simulink model "motor1"  (R2022b)
settings: Solver=ode45  StartTime=0.0  StopTime=5  MaxStep=0.0001  RelTol=1e-3
values from neighbouring files (symbols this model uses):
  Beq = 1.26e-6    (= 1.26e-06)    [ex1.m]    (also in ex2.m)
  Jeq = mot.J + mld.J / gbox.N^2    [ex1.m]    (also in ex2.m)
  tausf = 1e-2    (= 0.01)    [ex1.m]    (also in ex2.m)
undefined symbols (not defined in the file or in its folder): awu, dac, degs2rpm, diff, drv, gbox, mot, pid, rads2rpm, rpm2rads, sens, step
settings Model: Creator=loren  LastModifiedBy=loren
settings DataIOCC: ReturnWorkspaceOutputs=off
settings ModelReferenceCC: EnableRefExpFcnMdlSchedulingChecks=on

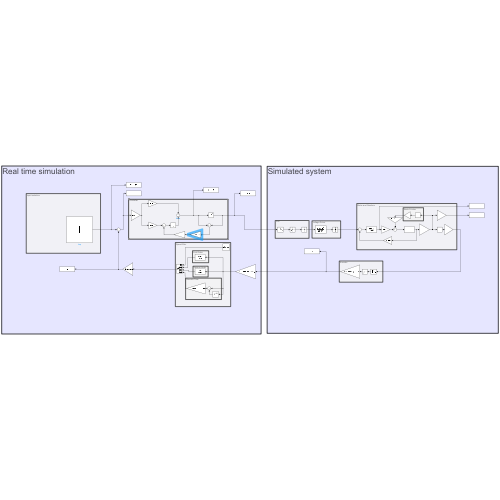
[thumbnail: Simulink's stored preview of the top-level diagram]
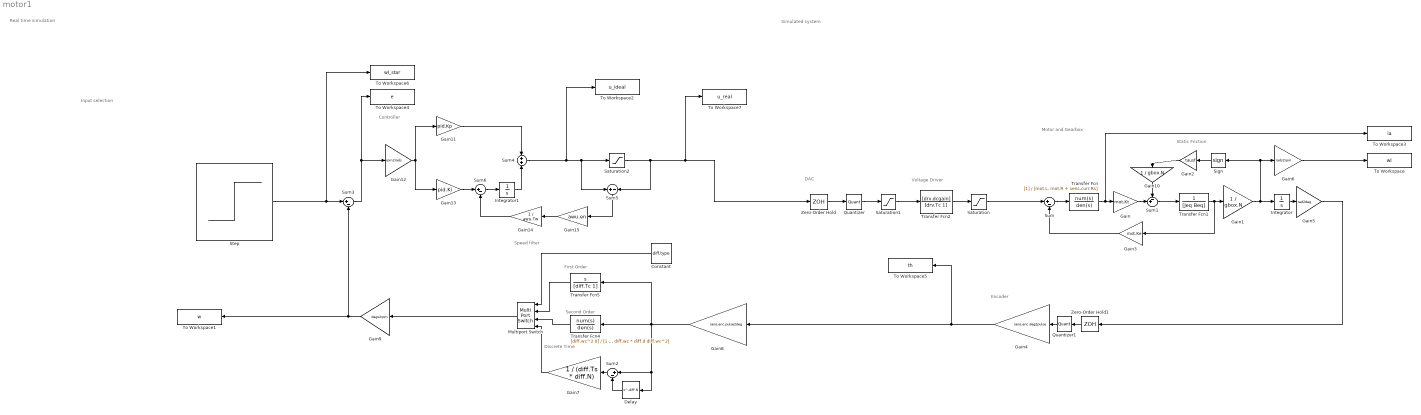
== system motor1 ==
  note: Simulated system
  note: Real time simulation
  note: Input selection
  note: Controller
  note: Speed filter
  note: Motor and Gearbox
  note: Discrete Time
  note: Second Order
  note: First Order
  note: Encoder
  note: DAC
  note: Voltage Driver
  note: Static Friction
  Constant : Constant  Value=diff.type
  Delay : Delay  DelayLength=diff.N
  Gain : Gain  Gain=mot.Kt
  Gain1 : Gain  Gain=1 / gbox.N
  Gain10 : Gain  Gain=1 / gbox.N
  Gain11 : Gain  Gain=pid.Kp
  Gain12 : Gain  Gain=rpm2rads
  Gain13 : Gain  Gain=pid.Ki
  Gain14 : Gain  Gain=1 / awu.Tw
  Gain15 : Gain  Gain=awu.en
  Gain2 : Gain  Gain=tausf
  Gain3 : Gain  Gain=mot.Ke
  Gain4 : Gain  Gain=sens.enc.deg2pulse
  Gain5 : Gain  Gain=rad2deg
  Gain6 : Gain  Gain=rads2rpm
  Gain7 : Gain  Gain=1 / (diff.Ts * diff.N)
  Gain8 : Gain  Gain=sens.enc.pulse2deg
  Gain9 : Gain  Gain=degs2rpm
  Integrator : Integrator
  Integrator1 : Integrator
  Multiport Switch : MultiPortSwitch  SaturateOnIntegerOverflow=off  InputSameDT=off
  Quantizer : Quantizer  QuantizationInterval=dac.q
  Quantizer1 : Quantizer  QuantizationInterval=sens.enc.pulse2deg
  Saturation : Saturate  UpperLimit=drv.outmax  LowerLimit=-drv.outmax
  Saturation1 : Saturate  UpperLimit=dac.V  LowerLimit=-dac.V
  Saturation2 : Saturate  UpperLimit=dac.V  LowerLimit=-dac.V
  Sign : Signum  ZeroCross=off
  Step : Step  Time=step.T  After=step.A  SampleTime=0
  Sum{,2..3,6} (4 alike) : Sum  Inputs=|+-
  Sum1 : Sum  Inputs=-+|
  Sum4 : Sum  Inputs=+|+
  Sum5 : Sum  Inputs=+|-
  To Workspace : ToWorkspace  VariableName=wl  SaveFormat=Timeseries  SampleTime=-1
  To Workspace1 : ToWorkspace  VariableName=w  SaveFormat=Timeseries  SampleTime=-1
  To Workspace2 : ToWorkspace  VariableName=u_ideal  SaveFormat=Timeseries  SampleTime=-1
  To Workspace3 : ToWorkspace  VariableName=ia  SaveFormat=Timeseries  SampleTime=-1
  To Workspace4 : ToWorkspace  VariableName=e  SaveFormat=Timeseries  SampleTime=-1
  To Workspace5 : ToWorkspace  VariableName=th  SaveFormat=Timeseries  SampleTime=-1
  To Workspace6 : ToWorkspace  VariableName=wl_star  SaveFormat=Timeseries  SampleTime=-1
  To Workspace7 : ToWorkspace  VariableName=u_real  SaveFormat=Timeseries  SampleTime=-1
  Transfer Fcn : TransferFcn  Denominator=[mot.L, mot.R + sens.curr.Rs]
  Transfer Fcn1 : TransferFcn  Denominator=[Jeq Beq]
  Transfer Fcn2 : TransferFcn  Numerator=[drv.dcgain]  Denominator=[drv.Tc 1]
  Transfer Fcn4 : TransferFcn  Numerator=[diff.wc^2 0]  Denominator=[1 2 * diff.wc * diff.d diff.wc^2]
  Transfer Fcn5 : TransferFcn  Numerator=[1 0]  Denominator=[diff.Tc 1]
  Zero-Order Hold : ZeroOrderHold  SampleTime=dac.Ts
  Zero-Order Hold1 : ZeroOrderHold  SampleTime=dac.Ts
  wires:
  Gain/1 -> Sum1/2
  Transfer Fcn/1 -> To Workspace3/1, Gain/1
  Sum/1 -> Transfer Fcn/1
  Saturation/1 -> Sum/1
  Transfer Fcn1/1 -> Gain3/1, Gain1/1
  Sum1/1 -> Transfer Fcn1/1
  Gain3/1 -> Sum/2
  Gain2/1 -> Gain10/1
  Gain1/1 -> Integrator/1, Gain6/1, Sign/1
  Sign/1 -> Gain2/1
  Integrator/1 -> Gain5/1
  Gain6/1 -> To Workspace/1
  Transfer Fcn2/1 -> Saturation/1
  Saturation1/1 -> Transfer Fcn2/1
  Zero-Order Hold/1 -> Quantizer/1
  Quantizer/1 -> Saturation1/1
  Zero-Order Hold1/1 -> Quantizer1/1
  Quantizer1/1 -> Gain4/1
  Gain4/1 -> To Workspace5/1, Gain8/1
  Gain5/1 -> Zero-Order Hold1/1
  Gain8/1 -> Transfer Fcn5/1, Transfer Fcn4/1, Delay/1, Sum2/1
  Delay/1 -> Sum2/2
  Sum2/1 -> Gain7/1
  Multiport Switch/1 -> Gain9/1
  Transfer Fcn5/1 -> Multiport Switch/2
  Transfer Fcn4/1 -> Multiport Switch/3
  Constant/1 -> Multiport Switch/1
  Gain9/1 -> To Workspace1/1, Sum3/2
  Sum3/1 -> Gain12/1, To Workspace4/1
  Gain10/1 -> Sum1/1
  Gain12/1 -> Gain11/1, Gain13/1
  Sum4/1 -> Saturation2/1, Sum5/1, To Workspace2/1
  Gain11/1 -> Sum4/1
  Integrator1/1 -> Sum4/2
  Gain7/1 -> Multiport Switch/4
  Step/1 -> To Workspace6/1, Sum3/1
  Gain13/1 -> Sum6/1
  Sum6/1 -> Integrator1/1
  Saturation2/1 -> Sum5/2, To Workspace7/1, Zero-Order Hold/1
  Sum5/1 -> Gain15/1
  Gain14/1 -> Sum6/2
  Gain15/1 -> Gain14/1
